simulink model "inverted_double_pendulum_on_a_cart_model_lin"  (R2019b)
settings: Solver=ode45  StartTime=0.0  StopTime=10  RelTol=1e-3  EnableMultiTasking=on
PreLoadFcn:
  | inverted_double_pendulum_on_a_cart
InitFcn:
  | inverted_double_pendulum_on_a_cart
StartFcn:
  | inverted_double_pendulum_on_a_cart
values from neighbouring files (symbols this model uses):
  A = [0 0 0 0 ((-m2)*g*m1-m1^2*g)/(m1*m0) 0 ... (first row only)    [inverted_double_pendulum_on_a_cart.m]
  B = [1 -1/l1 0 0 0 0]'    [inverted_double_pendulum_on_a_cart.m]
  C = eye(6)    [inverted_double_pendulum_on_a_cart.m]
  initial_conditions = [x theta1 theta2 x_dot theta1_dot theta2_dot]    [inverted_double_pendulum_on_a_cart.m]
  K = lqr(sys, Q, R)    [inverted_double_pendulum_on_a_cart.m]
settings Model: Creator=Nabeel  LastModifiedBy=Eugene
settings DataIOCC: LimitDataPoints=on  SaveFormat=Array  ReturnWorkspaceOutputs=off
settings OptimizationCC: LifeSpan=inf
settings DebuggingCC: SFUnexpectedBacktrackingDiag=warning  SFNoUnconditionalDefaultTransitionDiag=warning  SFExecutionAtInitializationDiag=none  ArithmeticOperatorsInVariantConditions=warning
settings HardwareCC: ProdBitPerPointer=32  ProdBitPerSizeT=32  ProdBitPerPtrDiffT=32  ProdLargestAtomicFloat=None  ProdIntDivRoundTo=Undefined  ProdEndianess=Unspecified  ProdWordSize=32  ProdHWDeviceType=32-bit Generic
settings ModelReferenceCC: PropagateSignalLabelsOutOfModel=off
settings SFSimCC: SimUseLocalCustomCode=off  CustomCodeUndefinedFunction=UseInterfaceOnly
settings RTWCC: RTWUseLocalCustomCode=off
settings CodeAppCC: StateflowObjectComments=on
settings GRTTargetCC: TargetLangStandard=C89/C90 (ANSI)  GeneratePreprocessorConditionals=Disable all
settings ConfigComp: CovMetricSettings=dw  CovHtmlReporting=on  CovSaveCumulativeToWorkspaceVar=on  CovSaveSingleToWorkspaceVar=on  CovExternalEMLEnable=off

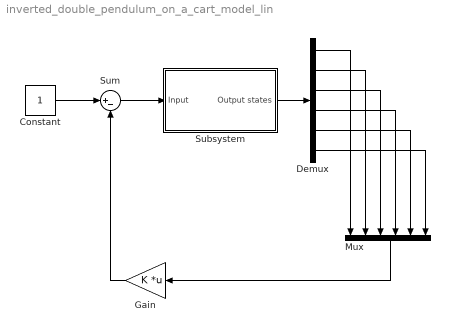
== system inverted_double_pendulum_on_a_cart_model_lin ==
  Constant : Constant
  Demux : Demux  Outputs=6
  Gain : Gain  Gain=K  Multiplication=Matrix(K*u)
  Mux : Mux  Inputs=6
  Subsystem : Subsystem
  Sum : Sum  Inputs=|+-
  wires:
  Sum/1 -> Subsystem/1(Input)
  Demux/3 -> Mux/3
  Mux/1 -> Gain/1
  Demux/1 -> Mux/1
  Demux/5 -> Mux/5
  Demux/2 -> Mux/2
  Demux/4 -> Mux/4
  Demux/6 -> Mux/6
  Constant/1 -> Sum/1
  Subsystem/1(Output states) -> Demux/1
  Gain/1 -> Sum/2

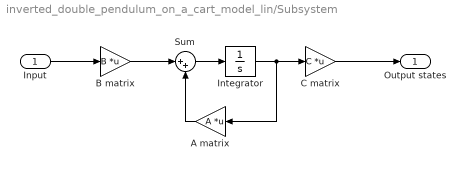
== system inverted_double_pendulum_on_a_cart_model_lin/Subsystem ==
  Input : Inport
  A matrix : Gain  Gain=A  Multiplication=Matrix(K*u)
  B matrix : Gain  Gain=B  Multiplication=Matrix(K*u)
  C matrix : Gain  Gain=C  Multiplication=Matrix(K*u)
  Integrator : Integrator  InitialCondition=initial_conditions
  Sum : Sum  Inputs=|++
  Output states : Outport
  wires:
  Input/1 -> B matrix/1
  C matrix/1 -> Output states/1
  B matrix/1 -> Sum/1
  Integrator/1 -> C matrix/1, A matrix/1
  Sum/1 -> Integrator/1
  A matrix/1 -> Sum/2
